simulink model "BLDCctrlBasedOnMBDPILtop"  (R2020b)
settings: Solver=FixedStepDiscrete  StartTime=0.0  StopTime=inf  FixedStep=1e-6  RelTol=1e-3
PreLoadFcn:
  | load('structMBDMotorCrtl.mat');
libraries: powerlib x10, powerlib_meascontrol x3
settings Model: Creator=k  LastModifiedBy=k

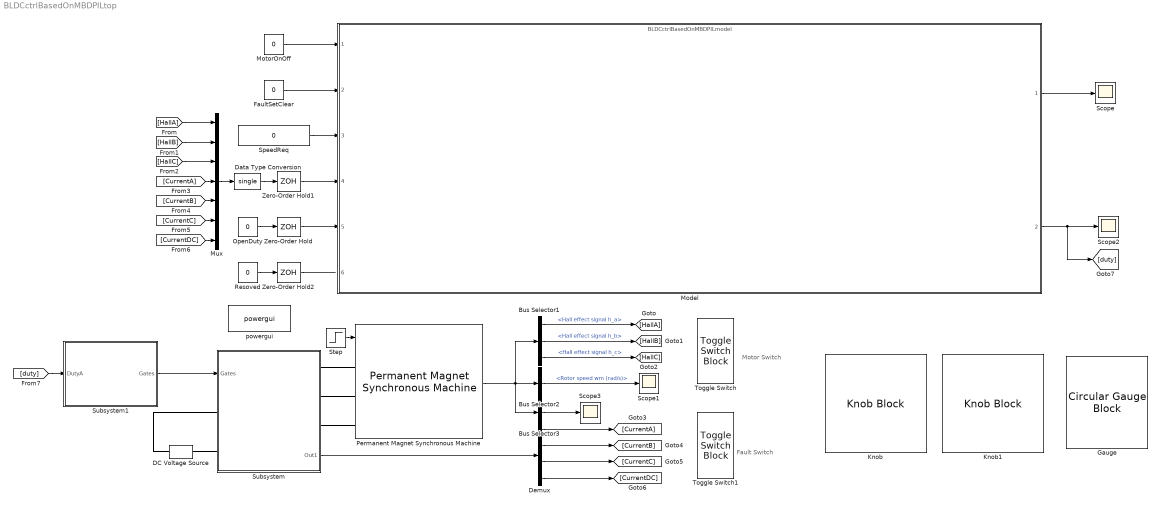
== system BLDCctrlBasedOnMBDPILtop ==
  note: Fault Switch
  note: Motor Switch
  Bus Selector1 : BusSelector  OutputSignals=Hall effect signal h_a,Hall effect signal h_b,Hall effect signal h_c
  Bus Selector2 : BusSelector  OutputSignals=Rotor speed wm (rad/s)
  Bus Selector3 : BusSelector  OutputSignals=Stator current is_a (A),Stator current is_b (A),Stator current is_c (A)  OutputAsBus=on
  DC Voltage Source : powerlib/Electrical Sources/DC Voltage Source  Amplitude=200  Measurements=None
  Data Type Conversion : DataTypeConversion  OutDataTypeStr=single
  Demux : Demux
  FaultSetClear : Constant  Value=0  OutDataTypeStr=boolean
  Gauge : CircularGaugeBlock  ScaleMax=150
  Knob : KnobBlock  TickInterval=20
  Knob1 : KnobBlock  ScaleMax=1  TickInterval=0.2
  Model : ModelReference  ModelNameDialog=BLDCctrlBasedOnMBDPILmodel.slx  SimulationMode=Processor-in-the-loop (PIL)  ModelReferenceVersion=1.113
  MotorOnOff : Constant  Value=0  OutDataTypeStr=boolean
  Mux : Mux  Inputs=7
  OpenDuty : Constant  Value=0  OutDataTypeStr=single
  Permanent Magnet Synchronous Machine : powerlib/Machines/Permanent Magnet Synchronous Machine  NbPhases=3  FluxDistribution=Trapezoidal  RotorType=Round  MechanicalLoad=Torque Tm  PresetModel=No  ShowDetailedParameters=on  MeasurementBus=off  Resistance=2.8750  Inductance=8.5e-3  dqInductances=[8.5e-3, 8.5e-3]  La=0.000835  MachineConstant=Flux linkage established by magnets (V.s)  Flux=0.175  VoltageCst=146.6077  TorqueCst=1.4  Flat=120  Mechanical=[ 0.8e-3, 1e-3 4]  PolePairs=4  InitialConditions=[0,0, 0,0]  InitialConditions5ph=[0 0 0 0 0 0]  RefAngle=90 degrees behind phase A axis (modified Park)  IterativeDiscreteModel=Trapezoidal non iterative  TsBlock=-1  TsPowergui=0
  Resoved : Constant  Value=0  OutDataTypeStr=single
  Scope{,1..3} (4 alike) : Scope
  SpeedReq : Constant  Value=0  OutDataTypeStr=single
  Step : Step  Time=0.25  SampleTime=0
  Subsystem : Subsystem
      settings: PortSchema="{\"entries\":[{\"content\":{\"sides\":[{\"content\":{\"connectorIds\":[\"In1\",\"LConn1\",\"LConn2\"]},\"type\":\"ConnectorPlacement.EquallySpacedRectSide\",\"uuid\":\"3e830c6c-b48e-4079-a555-63399f867b77\"},{\"content\":{\"connectorIds\":[\"RConn1\",\"RConn2\",\"RConn3\",\"Out1\"],\"side\":\"RIGHT\"},\"type\":\"ConnectorPlacement.EquallySpacedRectSide\",\"uuid\":\"e14bd0c3-2e36-4f0a-b270-beb41da57375\"},{\"content\":{\"connectorIds\":[],\"side\":\"TOP\"},\"type\":\"ConnectorPlacement.EquallySpacedRectSide\",\"uuid\":\"09179360-9fc0-4e49-92b5-7039012dd2c1\"},{\"content\":{\"connectorIds\":[],\"side\":\"HIDDEN\"},\"type\":\"ConnectorPlacement.EquallySpacedRectSide\",\"uuid\":\"af73253b-f07c-4a33-82ef-931e630f0fb0\"}]},\"type\":\"ConnectorPlacement.EquallySpacedConnector\",\"uuid\":\"7ce09c9c-6d00-4ec6-ad58-4c4a30439337\"}],\"packageUris\":[\"http://schema.mathworks.com/mf0/Connector/R2020b\"],\"version\":\"1.0\"}"
  Subsystem1 : Subsystem
  Toggle Switch : ToggleSwitchBlock  LabelPosition=Hide
      settings: Values={{'Off', 'On'}, [0 1]}
  Toggle Switch1 : ToggleSwitchBlock  LabelPosition=Hide
      settings: Values={{'Off', 'On'}, [0 1]}
  Zero-Order Hold : ZeroOrderHold  SampleTime=0.0001
  Zero-Order Hold1 : ZeroOrderHold  SampleTime=0.0001
  Zero-Order Hold2 : ZeroOrderHold  SampleTime=0.0001
  powergui : powerlib/powergui  Priority=2  SimulationMode=Discrete  SampleTime=1e-6  frequency=60  Iterations=50  frequencyindice=0  Pbase=100e6  ErrMax=1e-4  UnitsV=kV  UnitsW=MW  buscounter=0  FunctionMessages=off  echomessages=off  EnableUseOfTLC=off  CurrentSourceSwitches=off  DisableSnubberDevices=off  DisableRonSwitches=off  DisableVfSwitches=off  DisplayEquations=off  AutomaticDiscreteSolvers=off  SolverType=Tustin/Backward Euler (TBE)  Interpol=off  ExternalGateDelay=off  methode=off  Ts=0  x0status=blocks  SPID=off  SwTol=0  HookPort=off  NonlinearTolerance=1e-4  nMaxIteration=100  ContinueOnMaxIteration=off  RestoreLinks=warning  ResistiveCurrentMeasurement=off  Frange=[0:2:500]  Ylog=off  Xlog=on  ShowGrid=off  save=off  variable=ZData  structure=0  ZoomFFT=on  StartTime=0.0  cycles=1  DisplayStyle=1  fundamental=60  FreqAxis=off  MaxFrequency=1000  frequencyindicesteady=1  RmsSteady=1  display=off
  wires:
  MotorOnOff/1 -> Model/1
  FaultSetClear/1 -> Model/2
  Bus Selector2/1 -> Scope1/1  "<Rotor speed wm (rad/s)>"
  Bus Selector3/1 -> Scope3/1
  Subsystem/1(Out1) -> Demux/1
  Step/1 -> Permanent Magnet Synchronous Machine/1
  Permanent Magnet Synchronous Machine/1 -> Bus Selector1/1, Bus Selector2/1, Bus Selector3/1
  Bus Selector1/1 -> [HallA]  "<Hall effect signal h_a>"
  Bus Selector1/2 -> [HallB]  "<Hall effect signal h_b>"
  Bus Selector1/3 -> [HallC]  "<Hall effect signal h_c>"
  Demux/1 -> [CurrentA]
  Demux/4 -> [CurrentDC]
  Demux/2 -> [CurrentB]
  Demux/3 -> [CurrentC]
  SpeedReq/1 -> Model/3
  OpenDuty/1 -> Zero-Order Hold/1
  Model/1 -> Scope/1
  Model/2 -> Scope2/1, [duty]
  [CurrentA] -> Mux/4
  [CurrentB] -> Mux/5
  [CurrentC] -> Mux/6
  [CurrentDC] -> Mux/7
  [HallC] -> Mux/3
  [HallB] -> Mux/2
  [HallA] -> Mux/1
  Mux/1 -> Data Type Conversion/1
  Data Type Conversion/1 -> Zero-Order Hold1/1
  Zero-Order Hold/1 -> Model/5
  Zero-Order Hold1/1 -> Model/4
  Zero-Order Hold2/1 -> ?
  Resoved/1 -> Zero-Order Hold2/1
  Subsystem1/1(Gates) -> Subsystem/1(Gates)
  [duty] -> Subsystem1/1(DutyA)
  connections:
  DC Voltage Source/LConn1 -- Subsystem/LConn2
  DC Voltage Source/RConn1 -- Subsystem/LConn1
  Subsystem/RConn3 -- Permanent Magnet Synchronous Machine/LConn3
  Subsystem/RConn1 -- Permanent Magnet Synchronous Machine/LConn1
  Subsystem/RConn2 -- Permanent Magnet Synchronous Machine/LConn2

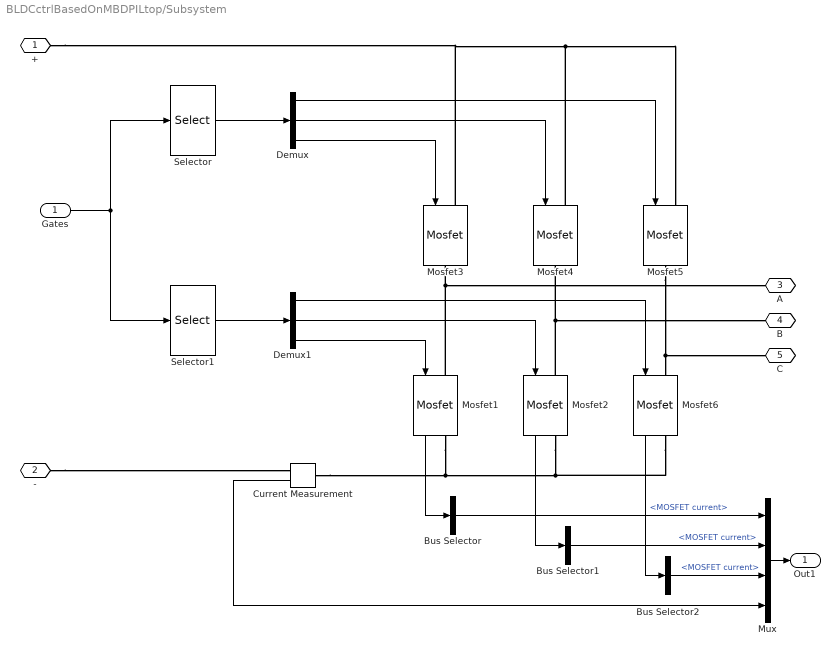
== system BLDCctrlBasedOnMBDPILtop/Subsystem ==
  Gates : Inport
  Bus Selector : BusSelector  OutputSignals=MOSFET current
  Bus Selector1 : BusSelector  OutputSignals=MOSFET current
  Bus Selector2 : BusSelector  OutputSignals=MOSFET current
  Current Measurement : powerlib/Measurements/Current Measurement  PhasorSimulation=off  OutputType=Complex  PSBequivalent=0
  Demux : Demux  Outputs=3
  Demux1 : Demux  Outputs=3
  Mosfet1 : powerlib/Power Electronics/Mosfet  Ron=0.001  Lon=0  Rd=0.0001  Vfd=0  IC=0  Rs=1e5  Cs=inf  Measurements=on
  Mosfet2 : powerlib/Power Electronics/Mosfet  Ron=0.001  Lon=0  Rd=0.0001  Vfd=0  IC=0  Rs=1e5  Cs=inf  Measurements=on
  Mosfet3 : powerlib/Power Electronics/Mosfet  Ron=0.001  Lon=0  Rd=0.0001  Vfd=0  IC=0  Rs=1e5  Cs=inf  Measurements=off
  Mosfet4 : powerlib/Power Electronics/Mosfet  Ron=0.001  Lon=0  Rd=0.0001  Vfd=0  IC=0  Rs=1e5  Cs=inf  Measurements=off
  Mosfet5 : powerlib/Power Electronics/Mosfet  Ron=0.001  Lon=0  Rd=0.0001  Vfd=0  IC=0  Rs=1e5  Cs=inf  Measurements=off
  Mosfet6 : powerlib/Power Electronics/Mosfet  Ron=0.001  Lon=0  Rd=0.0001  Vfd=0  IC=0  Rs=1e5  Cs=inf  Measurements=on
  Mux : Mux
  Selector : Selector  InputPortWidth=6  IndexOptions=Index vector (dialog)  Indices=[5 3 1]  OutputSizes=1
  Selector1 : Selector  InputPortWidth=6  IndexOptions=Index vector (dialog)  Indices=[6 4 2]  OutputSizes=1
  + : PMIOPort  Side=Left
  - : PMIOPort  Port=2  Side=Left
  A : PMIOPort  Port=3  Side=Right
  B : PMIOPort  Port=4  Side=Right
  C : PMIOPort  Port=5  Side=Right
  Out1 : Outport
  wires:
  Bus Selector1/1 -> Mux/2  "<MOSFET current>"
  Bus Selector2/1 -> Mux/3  "<MOSFET current>"
  Bus Selector/1 -> Mux/1  "<MOSFET current>"
  Mosfet1/1 -> Bus Selector/1
  Mosfet6/1 -> Bus Selector2/1
  Mosfet2/1 -> Bus Selector1/1
  Selector/1 -> Demux/1
  Gates/1 -> Selector/1, Selector1/1
  Current Measurement/1 -> Mux/4
  Mux/1 -> Out1/1
  Demux/1 -> Mosfet5/1
  Demux/2 -> Mosfet4/1
  Demux/3 -> Mosfet3/1
  Selector1/1 -> Demux1/1
  Demux1/3 -> Mosfet1/1
  Demux1/2 -> Mosfet2/1
  Demux1/1 -> Mosfet6/1
  connections:
  Mosfet2/LConn1 -- Mosfet4/RConn1 -- B/RConn1
  Mosfet1/RConn1 -- Current Measurement/LConn1 -- Mosfet2/RConn1 -- Mosfet6/RConn1
  Mosfet4/LConn1 -- Mosfet3/LConn1 -- +/RConn1 -- Mosfet5/LConn1
  Mosfet5/RConn1 -- C/RConn1 -- Mosfet6/LConn1
  Mosfet1/LConn1 -- A/RConn1 -- Mosfet3/RConn1
  -/RConn1 -- Current Measurement/RConn1

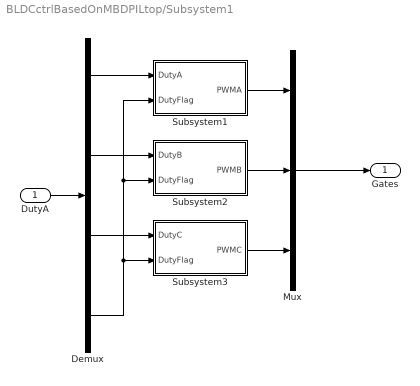
== system BLDCctrlBasedOnMBDPILtop/Subsystem1 ==
  DutyA : Inport
  Demux : Demux
  Mux : Mux  Inputs=3
  Subsystem1 : Subsystem
  Subsystem2 : Subsystem
  Subsystem3 : Subsystem
  Gates : Outport
  wires:
  Mux/1 -> Gates/1
  Subsystem1/1(PWMA) -> Mux/1
  Subsystem2/1(PWMB) -> Mux/2
  Subsystem3/1(PWMC) -> Mux/3
  Demux/2 -> Subsystem2/1(DutyB)
  Demux/3 -> Subsystem3/1(DutyC)
  Demux/4 -> Subsystem1/2(DutyFlag), Subsystem2/2(DutyFlag), Subsystem3/2(DutyFlag)
  DutyA/1 -> Demux/1
  Demux/1 -> Subsystem1/1(DutyA)

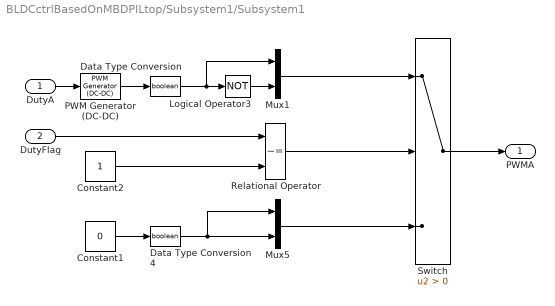
== system BLDCctrlBasedOnMBDPILtop/Subsystem1/Subsystem1 ==
  DutyA : Inport
  DutyFlag : Inport  Port=2
  Constant1 : Constant  Value=0
  Constant2 : Constant
  Data Type Conversion : DataTypeConversion  OutDataTypeStr=boolean
  Data Type Conversion4 : DataTypeConversion  OutDataTypeStr=boolean
  Logical Operator3 : Logic  Operator=NOT  AllPortsSameDT=off  OutDataTypeStr=boolean
  Mux1 : Mux  Inputs=2
  Mux5 : Mux  Inputs=2
  PWM Generator (DC-DC) : powerlib_meascontrol/Pulse & Signal Generators/PWM Generator (DC-DC)  Fsw=10000  Ts=1e-6
  Relational Operator : RelationalOperator  Operator=~=  OutDataTypeStr=boolean  RndMeth=Simplest
  Switch : Switch  Criteria=u2 > Threshold
  PWMA : Outport
  wires:
  Data Type Conversion/1 -> Logical Operator3/1, Mux1/1
  Mux1/1 -> Switch/1
  DutyA/1 -> PWM Generator (DC-DC)/1
  Mux5/1 -> Switch/3
  PWM Generator (DC-DC)/1 -> Data Type Conversion/1
  Constant1/1 -> Data Type Conversion4/1
  Logical Operator3/1 -> Mux1/2
  Data Type Conversion4/1 -> Mux5/2, Mux5/1
  Constant2/1 -> Relational Operator/2
  DutyFlag/1 -> Relational Operator/1
  Switch/1 -> PWMA/1
  Relational Operator/1 -> Switch/2

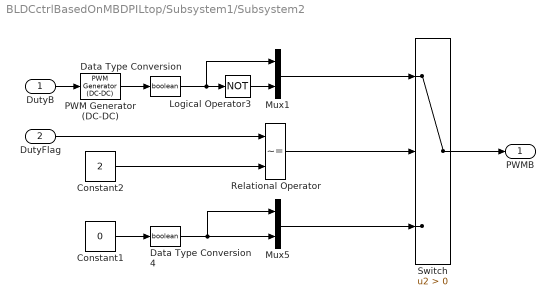
== system BLDCctrlBasedOnMBDPILtop/Subsystem1/Subsystem2 ==
  DutyB : Inport
  DutyFlag : Inport  Port=2
  Constant1 : Constant  Value=0
  Constant2 : Constant  Value=2
  Data Type Conversion : DataTypeConversion  OutDataTypeStr=boolean
  Data Type Conversion4 : DataTypeConversion  OutDataTypeStr=boolean
  Logical Operator3 : Logic  Operator=NOT  AllPortsSameDT=off  OutDataTypeStr=boolean
  Mux1 : Mux  Inputs=2
  Mux5 : Mux  Inputs=2
  PWM Generator (DC-DC) : powerlib_meascontrol/Pulse & Signal Generators/PWM Generator (DC-DC)  Fsw=10000  Ts=1e-6
  Relational Operator : RelationalOperator  Operator=~=  OutDataTypeStr=boolean  RndMeth=Simplest
  Switch : Switch  Criteria=u2 > Threshold
  PWMB : Outport
  wires:
  Relational Operator/1 -> Switch/2
  Switch/1 -> PWMB/1
  DutyFlag/1 -> Relational Operator/1
  Constant2/1 -> Relational Operator/2
  Data Type Conversion4/1 -> Mux5/1, Mux5/2
  Logical Operator3/1 -> Mux1/2
  Constant1/1 -> Data Type Conversion4/1
  PWM Generator (DC-DC)/1 -> Data Type Conversion/1
  Mux5/1 -> Switch/3
  DutyB/1 -> PWM Generator (DC-DC)/1
  Mux1/1 -> Switch/1
  Data Type Conversion/1 -> Mux1/1, Logical Operator3/1

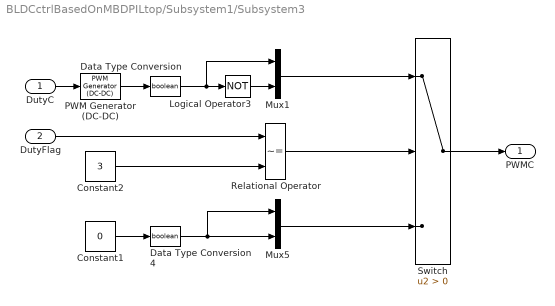
== system BLDCctrlBasedOnMBDPILtop/Subsystem1/Subsystem3 ==
  DutyC : Inport
  DutyFlag : Inport  Port=2
  Constant1 : Constant  Value=0
  Constant2 : Constant  Value=3
  Data Type Conversion : DataTypeConversion  OutDataTypeStr=boolean
  Data Type Conversion4 : DataTypeConversion  OutDataTypeStr=boolean
  Logical Operator3 : Logic  Operator=NOT  AllPortsSameDT=off  OutDataTypeStr=boolean
  Mux1 : Mux  Inputs=2
  Mux5 : Mux  Inputs=2
  PWM Generator (DC-DC) : powerlib_meascontrol/Pulse & Signal Generators/PWM Generator (DC-DC)  Fsw=10000  Ts=1e-6
  Relational Operator : RelationalOperator  Operator=~=  OutDataTypeStr=boolean  RndMeth=Simplest
  Switch : Switch  Criteria=u2 > Threshold
  PWMC : Outport
  wires:
  Data Type Conversion/1 -> Logical Operator3/1, Mux1/1
  Mux1/1 -> Switch/1
  DutyC/1 -> PWM Generator (DC-DC)/1
  Mux5/1 -> Switch/3
  PWM Generator (DC-DC)/1 -> Data Type Conversion/1
  Constant1/1 -> Data Type Conversion4/1
  Logical Operator3/1 -> Mux1/2
  Data Type Conversion4/1 -> Mux5/2, Mux5/1
  Constant2/1 -> Relational Operator/2
  DutyFlag/1 -> Relational Operator/1
  Switch/1 -> PWMC/1
  Relational Operator/1 -> Switch/2
